simulink model "FrameRotation"  (R2019a)
settings: Solver=ode15s  StartTime=0.0  StopTime=10  RelTol=1e-3
settings Model: Creator=paredis  LastModifiedBy=paredis
settings DataIOCC: SaveOutput=off  SaveTime=off

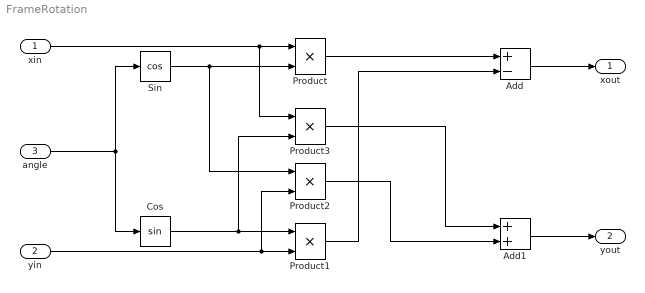
== system FrameRotation ==
  xin : Inport  OutDataTypeStr=double  PortDimensions=1  SampleTime=0
  yin : Inport  Port=2  OutDataTypeStr=double  PortDimensions=1  SampleTime=0
  angle : Inport  Port=3  OutDataTypeStr=double  PortDimensions=1
  Add : Sum  Inputs=+-
  Add1 : Sum
  Cos : Trigonometry
  Product{,1..3} (4 alike) : Product
  Sin : Trigonometry  Operator=cos
  xout : Outport  OutDataTypeStr=double  PortDimensions=1  SampleTime=0
  yout : Outport  Port=2  OutDataTypeStr=double  PortDimensions=1  SampleTime=0
  wires:
  Product1/1 -> Add/2
  Product3/1 -> Add1/1
  Cos/1 -> Product1/1, Product3/2
  yin/1 -> Product1/2, Product2/2
  Sin/1 -> Product/2, Product2/1
  Product/1 -> Add/1
  angle/1 -> Sin/1, Cos/1
  xin/1 -> Product3/1, Product/1
  Product2/1 -> Add1/2
  Add/1 -> xout/1
  Add1/1 -> yout/1
